simulink model "TestMdl"  (R2022b)
settings: Solver=VariableStepAuto  StartTime=0.0  StopTime=10.0  RelTol=1e-3
settings Model: Creator=rkaanth  LastModifiedBy=rkaanth

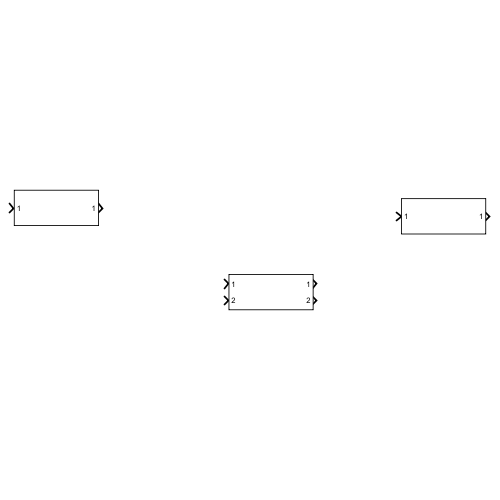
[thumbnail: Simulink's stored preview of the top-level diagram]
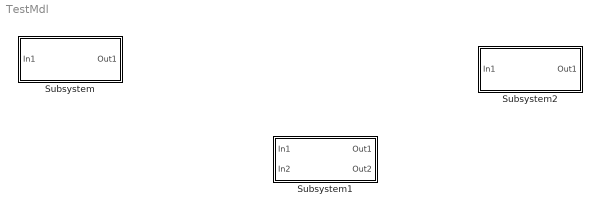
== system TestMdl ==
  Subsystem : Subsystem
  Subsystem1 : Subsystem
  Subsystem2 : Subsystem

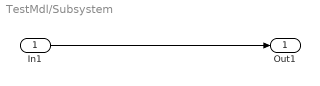
== system TestMdl/Subsystem ==
  In1 : Inport
  Out1 : Outport
  wires:
  In1/1 -> Out1/1

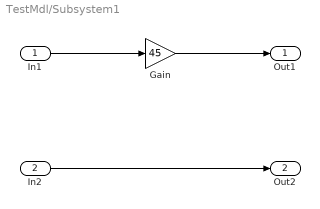
== system TestMdl/Subsystem1 ==
  In1 : Inport
  In2 : Inport  Port=2
  Gain : Gain  Gain=45
  Out1 : Outport
  Out2 : Outport  Port=2
  wires:
  In1/1 -> Gain/1
  Gain/1 -> Out1/1
  In2/1 -> Out2/1

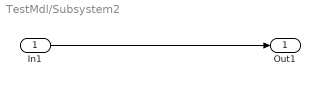
== system TestMdl/Subsystem2 ==
  In1 : Inport
  Out1 : Outport
  wires:
  In1/1 -> Out1/1
